simulink model "kukaslxctrl"  (R2016a)
settings: Solver=ode5  StartTime=0.0  StopTime=inf  FixedStep=.012  RelTol=1e-3
undefined symbols (not defined in the file or in its folder): Standard_Devices, UDP_Protocol
libraries: sldrtlib x2
settings Model: SimulationMode=external  Creator=julianleland  LastModifiedBy=julianleland
settings HardwareCC: ProdBitPerLong=64  ProdLargestAtomicFloat=None  ProdHWDeviceType=Intel->x86-64  TargetBitPerLong=64  TargetBitPerPointer=64  TargetIntDivRoundTo=Zero  TargetEndianess=LittleEndian  TargetWordSize=64  TargetHWDeviceType=Intel->x86-64
settings RTWCC: SystemTargetFile=sldrt.tlc  TemplateMakefile=sldrt.tmf  Description=Simulink Desktop Real-Time  RTWCompilerOptimization=on
settings CodeAppCC: MaxIdLength=95
settings SimulinkDesktopRealTimeCC: TargetPreCompLibLocation=C:\Program Files\MATLAB\R2016a\toolbox\sldrt\lib\win64  TargetLangStandard=C89/C90 (ANSI)  SupportVariableSizeSignals=off

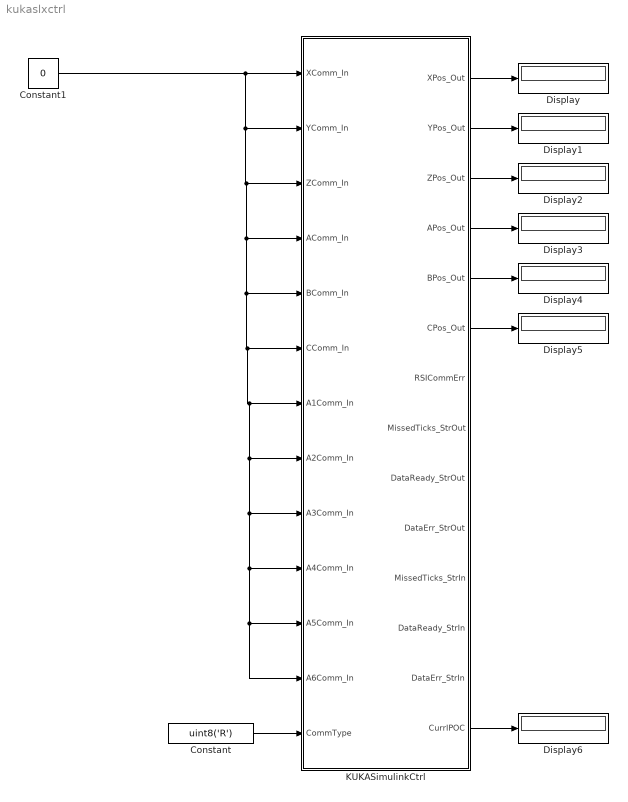
== system kukaslxctrl ==
  Constant : Constant  Value=uint8('R')
  Constant1 : Constant  Value=0
  Display{,1..6} (7 alike) : Display
  KUKASimulinkCtrl : Subsystem
  wires:
  KUKASimulinkCtrl/1(XPos_Out) -> Display/1
  KUKASimulinkCtrl/2(YPos_Out) -> Display1/1
  KUKASimulinkCtrl/3(ZPos_Out) -> Display2/1
  KUKASimulinkCtrl/4(APos_Out) -> Display3/1
  KUKASimulinkCtrl/5(BPos_Out) -> Display4/1
  KUKASimulinkCtrl/6(CPos_Out) -> Display5/1
  KUKASimulinkCtrl/14(CurrIPOC) -> Display6/1
  Constant/1 -> KUKASimulinkCtrl/13(CommType)
  Constant1/1 -> KUKASimulinkCtrl/12(A6Comm_In), KUKASimulinkCtrl/11(A5Comm_In), KUKASimulinkCtrl/10(A4Comm_In), KUKASimulinkCtrl/9(A3Comm_In), KUKASimulinkCtrl/8(A2Comm_In), KUKASimulinkCtrl/7(A1Comm_In), KUKASimulinkCtrl/6(CComm_In), KUKASimulinkCtrl/5(BComm_In), KUKASimulinkCtrl/4(AComm_In), KUKASimulinkCtrl/3(ZComm_In), KUKASimulinkCtrl/2(YComm_In), KUKASimulinkCtrl/1(XComm_In)

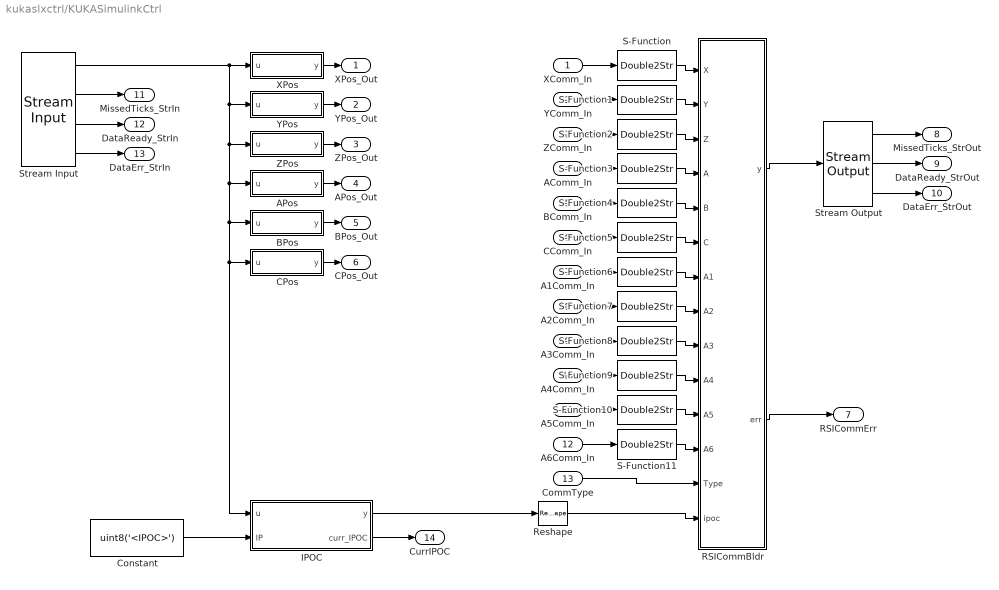
== system kukaslxctrl/KUKASimulinkCtrl ==
  XComm_In : Inport
  YComm_In : Inport  Port=2
  ZComm_In : Inport  Port=3
  AComm_In : Inport  Port=4
  BComm_In : Inport  Port=5
  CComm_In : Inport  Port=6
  A1Comm_In : Inport  Port=7
  A2Comm_In : Inport  Port=8
  A3Comm_In : Inport  Port=9
  A4Comm_In : Inport  Port=10
  A5Comm_In : Inport  Port=11
  A6Comm_In : Inport  Port=12
  CommType : Inport  Port=13
  APos : MATLAB Function  TreatAsAtomicUnit=on
  BPos : MATLAB Function  TreatAsAtomicUnit=on
  CPos : MATLAB Function  TreatAsAtomicUnit=on
  Constant : Constant  Value=uint8('<IPOC>')
  IPOC : MATLAB Function  TreatAsAtomicUnit=on
  RSICommBldr : MATLAB Function  TreatAsAtomicUnit=on
  Reshape : Reshape
  S-Function{,1..11} (12 alike) : S-Function  FunctionName=Double2Str  SFunctionDeploymentMode=off  EnableBusSupport=off
  Stream Input : sldrtlib/Stream Input  SampleTime=0.012  MaxMissedTicks=10  ShowMissedTicks=on  YieldWhenWaiting=on  DrvName=Standard_Devices/UDP_Protocol  DrvAddress=27277  DrvOptions=[174338148 53453]  DataTypes='238*uint16'  FormatString=repmat('%c',1,238)  Terminator='/Rob>'  ShowReady=on  ShowError=on
      settings: AttributesFormatString=Standard Devices\nUDP Protocol [6A8Dh]
  Stream Output : sldrtlib/Stream Output  SampleTime=0.012  MaxMissedTicks=10  ShowMissedTicks=on  YieldWhenWaiting=off  DrvName=Standard_Devices/UDP_Protocol  DrvAddress=27277  DrvOptions=[174338148 53453]  PortSizes=303  FormatString=repmat('%c',1,303)  ShowReady=on  ShowError=on  InitialValue=[]  FinalValue=[]
      settings: AttributesFormatString=Standard Devices\nUDP Protocol [6A8Dh]
  XPos : MATLAB Function  TreatAsAtomicUnit=on
  YPos : MATLAB Function  TreatAsAtomicUnit=on
  ZPos : MATLAB Function  TreatAsAtomicUnit=on
  XPos_Out : Outport
  YPos_Out : Outport  Port=2
  ZPos_Out : Outport  Port=3
  APos_Out : Outport  Port=4
  BPos_Out : Outport  Port=5
  CPos_Out : Outport  Port=6
  RSICommErr : Outport  Port=7
  MissedTicks_StrOut : Outport  Port=8
  DataReady_StrOut : Outport  Port=9
  DataErr_StrOut : Outport  Port=10
  MissedTicks_StrIn : Outport  Port=11
  DataReady_StrIn : Outport  Port=12
  DataErr_StrIn : Outport  Port=13
  CurrIPOC : Outport  Port=14
  wires:
  YComm_In/1 -> S-Function1/1
  BPos/1(y) -> BPos_Out/1
  CComm_In/1 -> S-Function5/1
  ZComm_In/1 -> S-Function2/1
  AComm_In/1 -> S-Function3/1
  BComm_In/1 -> S-Function4/1
  A6Comm_In/1 -> S-Function11/1
  RSICommBldr/2(err) -> RSICommErr/1
  A5Comm_In/1 -> S-Function10/1
  XPos/1(y) -> XPos_Out/1
  A2Comm_In/1 -> S-Function7/1
  A4Comm_In/1 -> S-Function9/1
  APos/1(y) -> APos_Out/1
  A3Comm_In/1 -> S-Function8/1
  YPos/1(y) -> YPos_Out/1
  A1Comm_In/1 -> S-Function6/1
  ZPos/1(y) -> ZPos_Out/1
  XComm_In/1 -> S-Function/1
  CPos/1(y) -> CPos_Out/1
  Stream Input/3 -> DataReady_StrIn/1
  S-Function/1 -> RSICommBldr/1(X)
  Stream Input/2 -> MissedTicks_StrIn/1
  Stream Input/1 -> IPOC/1(u), CPos/1(u), BPos/1(u), APos/1(u), ZPos/1(u), YPos/1(u), XPos/1(u)
  RSICommBldr/1(y) -> Stream Output/1
  IPOC/1(y) -> Reshape/1
  Constant/1 -> IPOC/2(IP)
  S-Function1/1 -> RSICommBldr/2(Y)
  S-Function2/1 -> RSICommBldr/3(Z)
  S-Function3/1 -> RSICommBldr/4(A)
  S-Function4/1 -> RSICommBldr/5(B)
  S-Function5/1 -> RSICommBldr/6(C)
  S-Function6/1 -> RSICommBldr/7(A1)
  S-Function7/1 -> RSICommBldr/8(A2)
  S-Function8/1 -> RSICommBldr/9(A3)
  S-Function9/1 -> RSICommBldr/10(A4)
  S-Function10/1 -> RSICommBldr/11(A5)
  S-Function11/1 -> RSICommBldr/12(A6)
  Stream Output/1 -> MissedTicks_StrOut/1
  Stream Output/2 -> DataReady_StrOut/1
  Stream Output/3 -> DataErr_StrOut/1
  Stream Input/4 -> DataErr_StrIn/1
  IPOC/2(curr_IPOC) -> CurrIPOC/1
  Reshape/1 -> RSICommBldr/14(ipoc)
  CommType/1 -> RSICommBldr/13(Type)

== matlab function kukaslxctrl/KUKASimulinkCtrl/XPos ==
  data: u input; y output
function y = fcn(u)
%#codegen

% Convert input into characters.
string = char(u);

% Locate start of X and Y strings
indx_X = strfind(string','X=');
indx_Y = strfind(string','Y=');

% Once X and Y strings have been located, grab the intervening characters
% (the X position). Otherwise, set to 0.
if ~isempty(indx_X)
    str_X = string((indx_X(1)+3):(indx_Y(1)-3));
    doub_X = str2double(str_X);
    y = doub_X;
else
    y = 0.0;
% TODO: Is this safe? Probably - if we're in abs mode and we command zero
% from some far distance away, it will cause a fault.
end

== matlab function kukaslxctrl/KUKASimulinkCtrl/RSICommBldr ==
  data: X input; Y input; Z input; A input; B input; C input; A1 input; A2 input; A3 input; A4 input; A5 input; A6 input; Type input; y output; ipoc input; err output
function [y, err] = fcn(X,Y,Z,A,B,C,A1,A2,A3,A4,A5,A6,Type,ipoc)
%#codegen

err = 0; % Default: define no error state.

%{
% Check whether we're inputting a RKorr or AKorr
switch Type
    case 82 % Either 'R' or 'r' passed in as uint8 - 82 or 114
        s1 = uint8('<Sen Type="ImFree"><RKorr ');
        s2 = uint8('X="');
        s3 = uint8('" Y="');
        s4 = uint8('" Z="');
        s5 = uint8('" A="');
        s6 = uint8('" B="');
        s7 = uint8('" C="');
        s8 = uint8('" /><IPOC>');
        s9 = uint8('</IPOC></Sen>');
        y = [s1 s2 X' s3 Y' s4 Z' s5 A' s6 B' s7 C' s8 ipoc' s9]
    case 65 % Either 'A' or 'a' passed in as uint8 - 65 or 97
        y = uint8('<Sen Type="ImFree"><RKorr '); % DUMMY - write correct string for analog input here instead
    otherwise
        y = uint8(''); % Send empty string so that KUKA gets upset
        err = 1; % Set error flag to 1
%}

crlf = [char(13) char(10)]; % Carriage return plus line feed
s1 = uint8(['<Sen Type="ImFree">' crlf]);
s1p1 = uint8(['<EStr></EStr>' crlf]);
s1p2 = uint8(['<Tech T21="1.09" T22="2.08" T23="3.07" T24="4.06" T25="5.05" T26="6.04" T27="7.03" T28="8.02" T29="9.01" T210="10.00" />' crlf]);
s1p3 = uint8('<RKorr ');
s2 = uint8('X="');
s3 = uint8('" Y="');
s4 = uint8('" Z="');
s5 = uint8('" A="');
s6 = uint8('" B="');
s7 = uint8('" C="');
s8 = uint8(['" />' crlf]);
s9 = uint8(['<DiO>125</DiO>' crlf]);
s10 = uint8('<IPOC>');
s11 = uint8(['</IPOC>' crlf]);
s12 = uint8('</Sen>');
%{
s8 = uint8('" /><IPOC>');
s9 = uint8('</IPOC><DiO>125</DiO></Sen>');
%}
y = [s1 s1p1 s1p2 s1p3 s2 X' s3 Y' s4 Z' s5 A' s6 B' s7 C' s8 s9 s10 ipoc' s11 s12];

end

== matlab function kukaslxctrl/KUKASimulinkCtrl/YPos ==
  data: u input; y output
function y = fcn(u)
%#codegen

% Convert input into characters.
string = char(u);

% Locate start of X and Y strings
indx_Y = strfind(string','Y=');
indx_Z = strfind(string','Z=');

% Once X and Y strings have been located, grab the intervening characters
% (the X position). Otherwise, set to 0.
if ~isempty(indx_Y)
    str_Y = string((indx_Y(1)+3):(indx_Z(1)-3));
    doub_Y = str2double(str_Y);
    y = doub_Y;
else
    y = 0.0;
% TODO: Is this safe? Probably - if we're in abs mode and we command zero
% from some far distance away, it will cause a fault.
end

== matlab function kukaslxctrl/KUKASimulinkCtrl/ZPos ==
  data: u input; y output
function y = fcn(u)
%#codegen

% Convert input into characters.
string = char(u);

% Locate start of X and Y strings
indx_Z = strfind(string','Z=');
indx_A = strfind(string','A=');

% Once X and Y strings have been located, grab the intervening characters
% (the X position). Otherwise, set to 0.
if ~isempty(indx_Z)
    str_Z = string((indx_Z(1)+3):(indx_A(1)-3));
    doub_Z = str2double(str_Z);
    y = doub_Z;
else
    y = 0.0;
% TODO: Is this safe? Probably - if we're in abs mode and we command zero
% from some far distance away, it will cause a fault.
end

== matlab function kukaslxctrl/KUKASimulinkCtrl/APos ==
  data: u input; y output
function y = fcn(u)
%#codegen

% Convert input into characters.
string = char(u);

% Locate start of X and Y strings
indx_A = strfind(string','A=');
indx_B = strfind(string','B=');

% Once X and Y strings have been located, grab the intervening characters
% (the X position). Otherwise, set to 0.
if ~isempty(indx_A)
    str_A = string((indx_A(1)+3):(indx_B(1)-3));
    doub_A = str2double(str_A);
    y = doub_A;
else
    y = 0.0;
% TODO: Is this safe? Probably - if we're in abs mode and we command zero
% from some far distance away, it will cause a fault.
end

== matlab function kukaslxctrl/KUKASimulinkCtrl/BPos ==
  data: u input; y output
function y = fcn(u)
%#codegen

% Convert input into characters.
string = char(u);

% Locate start of X and Y strings
indx_B = strfind(string','B=');
indx_C = strfind(string','C=');

% Once X and Y strings have been located, grab the intervening characters
% (the X position). Otherwise, set to 0.
if ~isempty(indx_B)
    str_B = string((indx_B(1)+3):(indx_C(1)-3));
    doub_B = str2double(str_B);
    y = doub_B;
else
    y = 0.0;
% TODO: Is this safe? Probably - if we're in abs mode and we command zero
% from some far distance away, it will cause a fault.
end

== matlab function kukaslxctrl/KUKASimulinkCtrl/CPos ==
  data: u input; y output
function y = fcn(u)
%#codegen

% Convert input into characters.
string = char(u);

% Locate start of X and Y strings
indx_C = strfind(string','C=');
indx_RSol = strfind(string','/><AIPos');

% Once X and Y strings have been located, grab the intervening characters
% (the X position). Otherwise, set to 0.
if ~isempty(indx_C)
    str_C = string((indx_C(1)+3):(indx_RSol(1)-3));
    doub_C = str2double(str_C);
    y = doub_C;
else
    y = 0.0;
% TODO: Is this safe? Probably - if we're in abs mode and we command zero
% from some far distance away, it will cause a fault.
end

== matlab function kukaslxctrl/KUKASimulinkCtrl/IPOC ==
  data: u input; y output; IP input; curr_IPOC output
function [y, curr_IPOC] = fcn(u, IP)
%#codegen

pos = 1;
pos_end = 2;
startStrLen = 6; % Length of IPOC start string. Hard-coded for speed
lenU = length(u);
%disp(['Reading input:' u']);

for i = 1:length(u)-startStrLen
    % Compare every set of 6 elements to IPOC start string. If their sum is
    % 6, we've found the start of the string.
    if (sum(u(i:i+(startStrLen-1)) == IP) == 6)
        pos = i+startStrLen;
    end
end

for i = pos:lenU
    if (u(i) == 60) % Search for next '<' character after IPOC
        pos_end = i-1;
        break; % Need to stop searching after we've found the end of the string
    end
end

% Pad IPOC with zeroes

ipocval = u(pos:pos_end);
ipoclen = length(ipocval);

ipoctemp = ones(1,8)*48;% zeros(1,10); % We may need to change this to ones(1,10)*48 if KUKA is looking for IPOC to be padded with zeroes before start.
for n = 7:-1:7-length(ipocval)+1
    ipoctemp(n) = ipocval(end-(7-n));
end

curr_IPOC = str2double(char(ipocval));
y = uint8(ipoctemp(1:7));
